simulink model "sim1"  (R2022b)
settings: Solver=VariableStepAuto  StartTime=0.0  StopTime=50  RelTol=1e-3
settings Model: Creator=ACER  LastModifiedBy=ACER

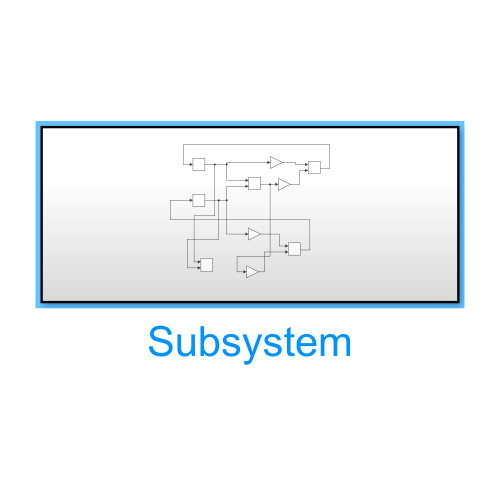
[thumbnail: Simulink's stored preview of the top-level diagram]
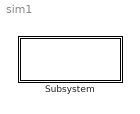
== system sim1 ==
  Subsystem : Subsystem

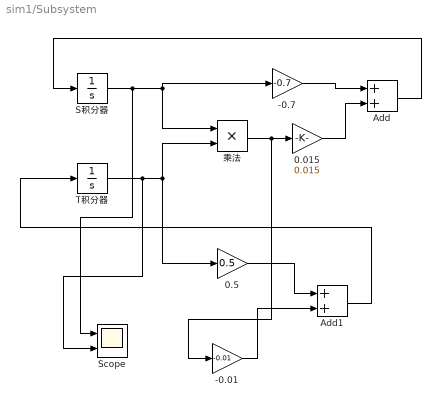
== system sim1/Subsystem ==
  -0.01 : Gain  Gain=-0.01
  -0.7 : Gain  Gain=-0.7
  0.015 : Gain  Gain=0.015
  0.5 : Gain  Gain=0.5
  Add : Sum
  Add1 : Sum
  Scope : Scope  NumInputPorts=2
  S积分器 : Integrator  InitialCondition=100
  T积分器 : Integrator  InitialCondition=100
  乘法 : Product
  wires:
  T积分器/1 -> Scope/2, 乘法/2, 0.5/1
  乘法/1 -> -0.01/1, 0.015/1
  0.015/1 -> Add/2
  -0.7/1 -> Add/1
  Add/1 -> S积分器/1
  0.5/1 -> Add1/1
  -0.01/1 -> Add1/2
  Add1/1 -> T积分器/1
  S积分器/1 -> Scope/1, 乘法/1, -0.7/1
